simulink model "simulationen"  (R2018b)
settings: Solver=VariableStepAuto  StartTime=0.0  StopTime=5  RelTol=1e-3
values from neighbouring files (symbols this model uses):
  b = 0.1    [handinTemplate.m]    (also in porte1.m; test.m)
  g = 9.82    [handinTemplate.m]    (also in porte1.m; test.m)
  I = 1/3*m*((2*l)^2)    (= 0.333333333333)    [porte1.m]    (also in test.m)
  l = 0.5    [handinTemplate.m]    (also in porte1.m; test.m)
  m = 1    [handinTemplate.m]    (also in porte1.m; test.m)
settings Model: Creator=Batman  LastModifiedBy=Batman

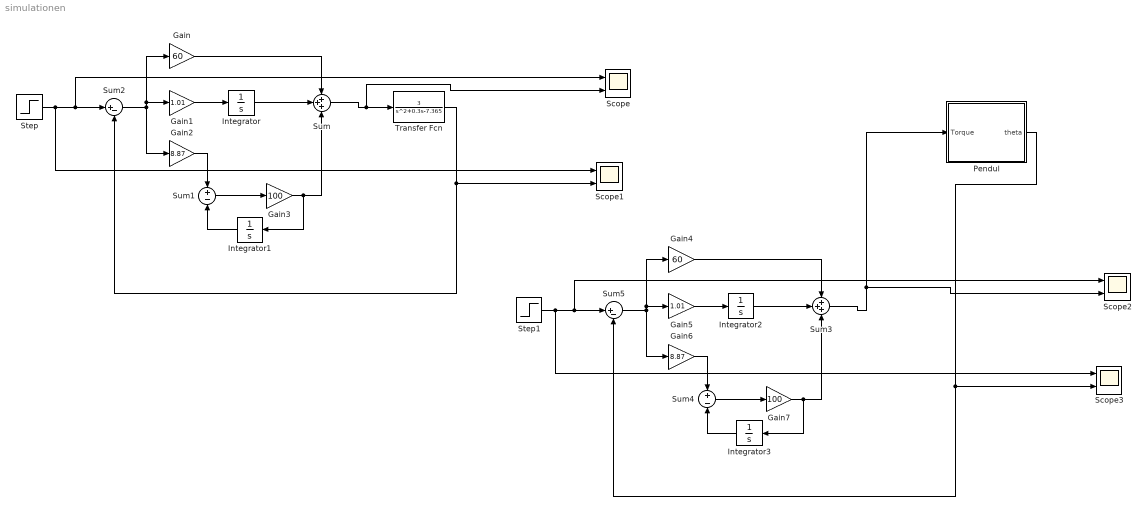
== system simulationen ==
  Gain : Gain  Gain=60
  Gain1 : Gain  Gain=1.01
  Gain2 : Gain  Gain=8.87
  Gain3 : Gain  Gain=100
  Gain4 : Gain  Gain=60
  Gain5 : Gain  Gain=1.01
  Gain6 : Gain  Gain=8.87
  Gain7 : Gain  Gain=100
  Integrator{,1..3} (4 alike) : Integrator
  Pendul : Subsystem
  Scope{,1..3} (4 alike) : Scope  NumInputPorts=2
  Step : Step  After=pi/3  SampleTime=0
  Step1 : Step  After=pi/3  SampleTime=0
  Sum : Sum  Inputs=+++
  Sum1 : Sum  Inputs=+-
  Sum2 : Sum  Inputs=|+-
  Sum3 : Sum  Inputs=+++
  Sum4 : Sum  Inputs=+-
  Sum5 : Sum  Inputs=|+-
  Transfer Fcn : TransferFcn  Numerator=[3]  Denominator=[1 0.3 -7.365]
  wires:
  Step/1 -> Scope1/1, Scope/1, Sum2/1
  Gain1/1 -> Integrator/1
  Gain/1 -> Sum/1
  Integrator/1 -> Sum/2
  Gain3/1 -> Sum/3, Integrator1/1
  Integrator1/1 -> Sum1/2
  Gain2/1 -> Sum1/1
  Sum1/1 -> Gain3/1
  Sum/1 -> Scope/2, Transfer Fcn/1
  Sum2/1 -> Gain1/1, Gain/1, Gain2/1
  Transfer Fcn/1 -> Scope1/2, Sum2/2
  Sum3/1 -> Pendul/1(Torque), Scope2/2
  Sum4/1 -> Gain7/1
  Gain5/1 -> Integrator2/1
  Gain6/1 -> Sum4/1
  Gain7/1 -> Sum3/3, Integrator3/1
  Integrator3/1 -> Sum4/2
  Integrator2/1 -> Sum3/2
  Pendul/1(theta) -> Scope3/2, Sum5/2
  Gain4/1 -> Sum3/1
  Sum5/1 -> Gain5/1, Gain4/1, Gain6/1
  Step1/1 -> Scope3/1, Scope2/1, Sum5/1

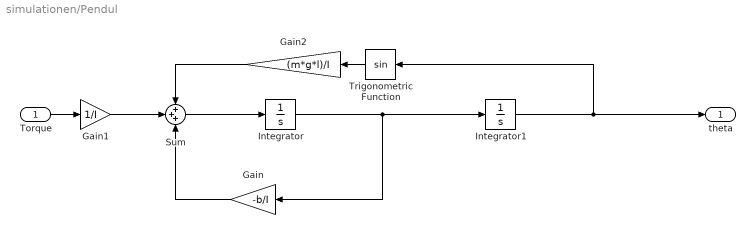
== system simulationen/Pendul ==
  Torque : Inport
  Gain : Gain  Gain=-b/I
  Gain1 : Gain  Gain=1/I
  Gain2 : Gain  Gain=(m*g*l)/I
  Integrator : Integrator
  Integrator1 : Integrator
  Sum : Sum  Inputs=+++
  Trigonometric Function : Trigonometry
  theta : Outport
  wires:
  Integrator1/1 -> Trigonometric Function/1, theta/1
  Sum/1 -> Integrator/1
  Torque/1 -> Gain1/1
  Gain1/1 -> Sum/2
  Gain2/1 -> Sum/1
  Gain/1 -> Sum/3
  Integrator/1 -> Gain/1, Integrator1/1
  Trigonometric Function/1 -> Gain2/1
